simulink model "RLCCircuit"  (R2020a)
settings: Solver=VariableStepAuto  StartTime=0.0  StopTime=50  RelTol=1e-3
settings Model: Creator=hp  LastModifiedBy=hp

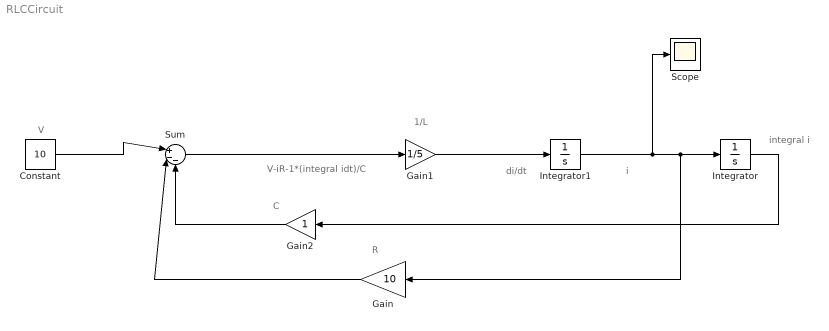
== system RLCCircuit ==
  note: integral i
  note: C
  note: 1/L
  note: V-iR-1*(integral idt)/C
  note: R
  note: V
  note: di/dt
  note: i
  Constant : Constant  Value=10
  Gain : Gain  Gain=10
  Gain1 : Gain  Gain=1/5
  Gain2 : Gain
  Integrator : Integrator
  Integrator1 : Integrator
  Scope : Scope
  Sum : Sum  Inputs=|+--
  wires:
  Sum/1 -> Gain1/1
  Constant/1 -> Sum/1
  Gain/1 -> Sum/2
  Gain1/1 -> Integrator1/1
  Gain2/1 -> Sum/3
  Integrator/1 -> Gain2/1
  Integrator1/1 -> Scope/1, Gain/1, Integrator/1
